simulink model "lateral_autopilot"  (R2018b)
settings: Solver=VariableStepAuto  StartTime=0.0  StopTime=250  RelTol=1e-3
values from neighbouring files (symbols this model uses):
  a_phi_1 = 2.87    [assignment2.m]
  a_phi_2 = -0.65    [assignment2.m]
  d = 1.5    [assignment2.m]
  g = 9.81    [assignment2.m]
  k_d_phi = 1.94    [assignment2.m]
  k_i_chi = 0.21    [assignment2.m]
  k_p_chi = 3.74    [assignment2.m]
  k_p_phi = -2    [assignment2.m]
  V_g = V_a    (= 580)    [assignment2.m]
settings Model: Creator=Magnus Dyre-Moe  LastModifiedBy=Magnus Dyre-Moe

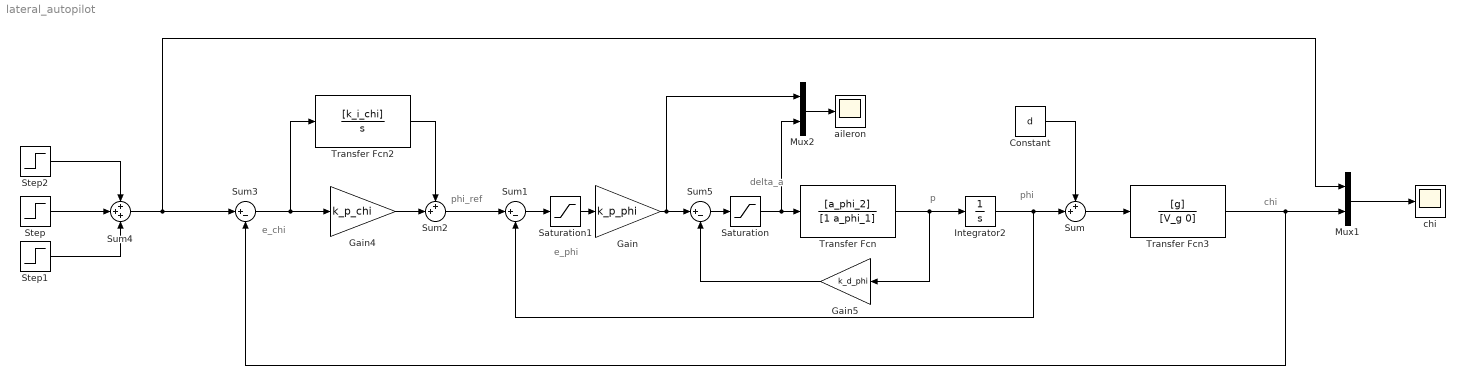
== system lateral_autopilot ==
  note: chi
  note: phi
  note: p
  note: delta_a
  note: e_phi
  note: phi_ref
  note: e_chi
  Constant : Constant  Value=d
  Gain : Gain  Gain=k_p_phi
  Gain4 : Gain  Gain=k_p_chi
  Gain5 : Gain  Gain=k_d_phi
  Integrator2 : Integrator
  Mux1 : Mux  Inputs=2
  Mux2 : Mux  Inputs=2
  Saturation : Saturate  UpperLimit=30  LowerLimit=-30
  Saturation1 : Saturate  UpperLimit=15  LowerLimit=-15
  Step : Step  Time=25  After=10  SampleTime=0
  Step1 : Step  Time=100  After=5  SampleTime=0
  Step2 : Step  Time=200  After=15  SampleTime=0
  Sum : Sum  Inputs=++|
  Sum1 : Sum  Inputs=|+-
  Sum2 : Sum  Inputs=++|
  Sum3 : Sum  Inputs=|+-
  Sum4 : Sum  Inputs=+++
  Sum5 : Sum  Inputs=|+-
  Transfer Fcn : TransferFcn  Numerator=[a_phi_2]  Denominator=[1 a_phi_1]
  Transfer Fcn2 : TransferFcn  Numerator=[k_i_chi]  Denominator=[1 0]
  Transfer Fcn3 : TransferFcn  Numerator=[g]  Denominator=[V_g 0]
  "aileron " : Scope
  chi : Scope
  wires:
  Sum5/1 -> Saturation/1
  Gain5/1 -> Sum5/2
  Transfer Fcn/1 -> Gain5/1, Integrator2/1
  Gain/1 -> Mux2/1, Sum5/1
  Sum2/1 -> Sum1/1
  Gain4/1 -> Sum2/2
  Transfer Fcn2/1 -> Sum2/1
  Sum3/1 -> Transfer Fcn2/1, Gain4/1
  Integrator2/1 -> Sum/2, Sum1/2
  Sum/1 -> Transfer Fcn3/1
  Transfer Fcn3/1 -> Mux1/2, Sum3/2
  Constant/1 -> Sum/1
  Saturation/1 -> Mux2/2, Transfer Fcn/1
  Sum1/1 -> Saturation1/1
  Saturation1/1 -> Gain/1
  Step1/1 -> Sum4/3
  Sum4/1 -> Mux1/1, Sum3/1
  Mux1/1 -> chi/1
  Step/1 -> Sum4/2
  Step2/1 -> Sum4/1
  Mux2/1 -> "aileron "/1
